simulink model "sampleModel134"  (Simulink 9.1)
settings: Solver=VariableStepAuto  StartTime=0.0  StopTime=10.0  RelTol=1e-3
undefined symbols (not defined in the file): DiscIntNeverNeededParam, Newton, Raphson
libraries: simulink x62
(part 1 of 2)
settings Model: Creator=DELL  LastModifiedBy=DELL
settings DataIOCC: SaveFormat=Dataset
settings OptimizationCC: LifeSpan=auto
settings DebuggingCC: UnderspecifiedInitializationDetection=Simplified  MergeDetectMultiDrivingBlocksExec=error  SFUnexpectedBacktrackingDiag=error  SFNoUnconditionalDefaultTransitionDiag=error  SFExecutionAtInitializationDiag=warning
settings HardwareCC: ProdBitPerPointer=64  ProdBitPerSizeT=64  ProdBitPerPtrDiffT=64  ProdLargestAtomicFloat=Float  ProdIntDivRoundTo=Zero  ProdEndianess=LittleEndian  ProdWordSize=64  ProdHWDeviceType=Intel->x86-64 (Windows64)
settings ModelReferenceCC: PropagateSignalLabelsOutOfModel=on
settings CodeAppCC: StateflowObjectComments=off
settings GRTTargetCC: TargetLangStandard=C99 (ISO)  CombineOutputUpdateFcns=on  GRTInterface=off
settings ConfigComp: CovMetricSettings=dwe  CovHtmlReporting=off  CovSaveCumulativeToWorkspaceVar=off  CovSaveSingleToWorkspaceVar=off  CovExternalEMLEnable=on

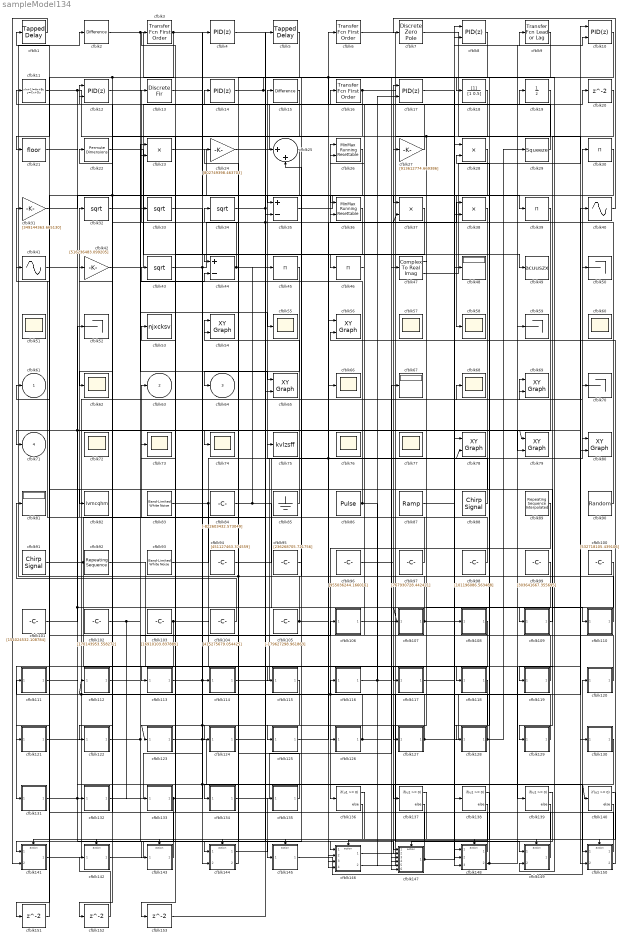
== system sampleModel134 ==
  cfblk1 : simulink/Discrete/Tapped Delay  vinit=0.0  samptime=-1  NumDelays=1  DelayOrder=Oldest  includeCurrent=off
  cfblk{8,10,12,17} (4 alike) : simulink/Continuous/PID Controller (2DOF)  Controller=PID  TimeDomain=Discrete-time  SampleTime=1  IntegratorMethod=Forward Euler  FilterMethod=Forward Euler  Form=Parallel  UseFilter=on  ControllerParametersSource=internal  P=1  I=1  D=0  N=100  b=1  c=1  InitialConditionSource=internal  InitialConditionForIntegrator=0  InitialConditionForFilter=0  ExternalReset=none  LimitOutput=off  UpperSaturationLimit=inf  LowerSaturationLimit=-inf  LinearizeAsGain=off  AntiWindupMode=none  Kb=1  TrackingMode=off  Kt=1  PParamMin=[]  PParamMax=[]  IParamMin=[]  IParamMax=[]  DParamMin=[]  DParamMax=[]  NParamMin=[]  NParamMax=[]  bParamMin=[]  bParamMax=[]  cParamMin=[]  cParamMax=[]  KbParamMin=[]  KbParamMax=[]  KtParamMin=[]  KtParamMax=[]  POutMin=[]  POutMax=[]  IOutMin=[]  IOutMax=[]  DOutMin=[]  DOutMax=[]  NOutMin=[]  NOutMax=[]  bOutMin=[]  bOutMax=[]  cOutMin=[]  cOutMax=[]  KbOutMin=[]  KbOutMax=[]  KtOutMin=[]  KtOutMax=[]  IntegratorOutMin=[]  IntegratorOutMax=[]  FilterOutMin=[]  FilterOutMax=[]  SumOutMin=[]  SumOutMax=[]  Sum1OutMin=[]  Sum1OutMax=[]  Sum2OutMin=[]  Sum2OutMax=[]  Sum3OutMin=[]  Sum3OutMax=[]  SumI1OutMin=[]  SumI1OutMax=[]  SumI2OutMin=[]  SumI2OutMax=[]  SumI3OutMin=[]  SumI3OutMax=[]  SumDOutMin=[]  SumDOutMax=[]  SaturationOutMin=[]  SaturationOutMax=[]  IntegratorContinuousStateAttributes=''  IntegratorStateMustResolveToSignalObject=off  IntegratorRTWStateStorageClass=Auto  FilterContinuousStateAttributes=''  FilterStateMustResolveToSignalObject=off  FilterRTWStateStorageClass=Auto  DifferentiatorICPrevScaledInput=0  DifferentiatorOutMin=[]  DifferentiatorOutMax=[]  FilterDiffOutCoefMin=[]  FilterDiffOutCoefMax=[]  SumDenOutMin=[]  SumDenOutMax=[]  SumNumOutMin=[]  SumNumOutMax=[]  ReciprocalOutMin=[]  ReciprocalOutMax=[]  DivideOutMin=[]  DivideOutMax=[]  TunerSelectOption=Transfer Function Based (PID Tuner App)
  cfblk100 : Constant  Value=[532718105.439106]  SampleTime=1
  cfblk101 : Constant  Value=[154024532.108784]  SampleTime=1
  cfblk102 : Constant  Value=[170143953.558272]  SampleTime=1
  cfblk103 : Constant  Value=[16910103.837889]  SampleTime=1
  cfblk104 : Constant  Value=[415275679.054425]  SampleTime=1
  cfblk105 : Constant  Value=[-179627298.961863]  SampleTime=1
  cfblk106 : Subsystem
  cfblk107 : Subsystem
  cfblk108 : Subsystem
  cfblk109 : Subsystem
  cfblk11 : DiscreteStateSpace
  cfblk110 : Subsystem
  cfblk111 : Subsystem
  cfblk112 : Subsystem
  cfblk113 : Subsystem
  cfblk114 : Subsystem
  cfblk115 : Subsystem
  cfblk116 : Subsystem
  cfblk117 : Subsystem
  cfblk118 : Subsystem
  cfblk119 : Subsystem
  cfblk120 : Subsystem
  cfblk121 : Subsystem
  cfblk122 : Subsystem
  cfblk123 : Subsystem
  cfblk124 : Subsystem
  cfblk125 : Subsystem
  cfblk126 : Subsystem
  cfblk127 : Subsystem
  cfblk128 : Subsystem
  cfblk129 : Subsystem
  cfblk13 : DiscreteFir  SampleTime=1
  cfblk130 : Subsystem
  cfblk131 : Subsystem
  cfblk132 : Subsystem
  cfblk133 : Subsystem
  cfblk134 : Subsystem
  cfblk135 : Subsystem
  cfblk{136..140} (5 alike) : If  IfExpression=u1 >= 0  SampleTime=1
  cfblk14 : simulink/Continuous/PID Controller  Controller=PID  TimeDomain=Discrete-time  SampleTime=1  IntegratorMethod=Forward Euler  FilterMethod=Forward Euler  Form=Parallel  UseFilter=on  ControllerParametersSource=internal  P=1  I=1  D=0  N=100  InitialConditionSource=internal  InitialConditionForIntegrator=0  InitialConditionForFilter=0  ExternalReset=none  LimitOutput=off  UpperSaturationLimit=inf  LowerSaturationLimit=-inf  LinearizeAsGain=off  AntiWindupMode=none  Kb=1  TrackingMode=off  Kt=1  PParamMin=[]  PParamMax=[]  IParamMin=[]  IParamMax=[]  DParamMin=[]  DParamMax=[]  NParamMin=[]  NParamMax=[]  KbParamMin=[]  KbParamMax=[]  KtParamMin=[]  KtParamMax=[]  POutMin=[]  POutMax=[]  IOutMin=[]  IOutMax=[]  DOutMin=[]  DOutMax=[]  NOutMin=[]  NOutMax=[]  KbOutMin=[]  KbOutMax=[]  KtOutMin=[]  KtOutMax=[]  IntegratorOutMin=[]  IntegratorOutMax=[]  FilterOutMin=[]  FilterOutMax=[]  SumOutMin=[]  SumOutMax=[]  SumI1OutMin=[]  SumI1OutMax=[]  SumI2OutMin=[]  SumI2OutMax=[]  SumI3OutMin=[]  SumI3OutMax=[]  SumDOutMin=[]  SumDOutMax=[]  SaturationOutMin=[]  SaturationOutMax=[]  IntegratorContinuousStateAttributes=''  IntegratorStateMustResolveToSignalObject=off  IntegratorRTWStateStorageClass=Auto  FilterContinuousStateAttributes=''  FilterStateMustResolveToSignalObject=off  FilterRTWStateStorageClass=Auto  DifferentiatorICPrevScaledInput=0  DifferentiatorOutMin=[]  DifferentiatorOutMax=[]  FilterDiffOutCoefMin=[]  FilterDiffOutCoefMax=[]  SumDenOutMin=[]  SumDenOutMax=[]  SumNumOutMin=[]  SumNumOutMax=[]  ReciprocalOutMin=[]  ReciprocalOutMax=[]  DivideOutMin=[]  DivideOutMax=[]  TunerSelectOption=Transfer Function Based (PID Tuner App)
  cfblk141 : Subsystem  TreatAsAtomicUnit=on
  cfblk142 : Subsystem  TreatAsAtomicUnit=on
  cfblk143 : Subsystem  TreatAsAtomicUnit=on
  cfblk144 : Subsystem  TreatAsAtomicUnit=on
  cfblk145 : Subsystem  TreatAsAtomicUnit=on
  cfblk146 : Subsystem  TreatAsAtomicUnit=on
  cfblk147 : Subsystem  TreatAsAtomicUnit=on
  cfblk148 : Subsystem  TreatAsAtomicUnit=on
  cfblk149 : Subsystem  TreatAsAtomicUnit=on
  cfblk15 : simulink/Discrete/Difference  ICPrevInput=0.0  OutMin=[]  OutMax=[]  OutDataTypeStr=Inherit: Inherit via back propagation  OutDataType=fixdt(1, 16)  OutScaling=2^-10  DoSatur=off
  cfblk150 : Subsystem  TreatAsAtomicUnit=on
  cfblk{20,151..153} (4 alike) : Delay  SampleTime=1
  cfblk16 : simulink/Discrete/Transfer Fcn First Order  PoleZ=0.95  ICPrevOutput=0.0  DoSatur=off
      settings: SourceProductName=Simulink
  cfblk18 : DiscreteFilter  SampleTime=1
  cfblk19 : UnitDelay
  cfblk2 : simulink/Discrete/Difference  ICPrevInput=0.0  OutMin=[]  OutMax=[]  OutDataTypeStr=Inherit: Inherit via back propagation  OutDataType=fixdt(1, 16)  OutScaling=2^-10  DoSatur=off
  cfblk21 : Rounding
  cfblk22 : PermuteDimensions
  cfblk23 : Product  Inputs=**
  cfblk24 : Gain  Gain=[802749398.463703]
  cfblk25 : Sum  Inputs=|++
  cfblk26 : simulink/Math Operations/MinMax Running Resettable  Function=min  vinit=0.0
  cfblk27 : Gain  Gain=[913612774.669386]
  cfblk28 : Product
  cfblk29 : Squeeze
  cfblk3 : simulink/Discrete/Transfer Fcn First Order  PoleZ=0.95  ICPrevOutput=0.0  DoSatur=off
      settings: SourceProductName=Simulink
  cfblk{30,39,45..46} (4 alike) : Product  Inputs=*
  cfblk31 : Gain  Gain=[349144363.665130]
  cfblk{32..34,43} (4 alike) : Sqrt  SaturateOnIntegerOverflow=on
  cfblk35 : Sum  Inputs=+-
  cfblk36 : simulink/Math Operations/MinMax Running Resettable  Function=min  vinit=0.0
  cfblk37 : Product
  cfblk38 : Product
  cfblk4 : simulink/Continuous/PID Controller  Controller=PID  TimeDomain=Discrete-time  SampleTime=1  IntegratorMethod=Forward Euler  FilterMethod=Forward Euler  Form=Parallel  UseFilter=on  ControllerParametersSource=internal  P=1  I=1  D=0  N=100  InitialConditionSource=internal  InitialConditionForIntegrator=0  InitialConditionForFilter=0  ExternalReset=none  LimitOutput=off  UpperSaturationLimit=inf  LowerSaturationLimit=-inf  LinearizeAsGain=off  AntiWindupMode=none  Kb=1  TrackingMode=off  Kt=1  PParamMin=[]  PParamMax=[]  IParamMin=[]  IParamMax=[]  DParamMin=[]  DParamMax=[]  NParamMin=[]  NParamMax=[]  KbParamMin=[]  KbParamMax=[]  KtParamMin=[]  KtParamMax=[]  POutMin=[]  POutMax=[]  IOutMin=[]  IOutMax=[]  DOutMin=[]  DOutMax=[]  NOutMin=[]  NOutMax=[]  KbOutMin=[]  KbOutMax=[]  KtOutMin=[]  KtOutMax=[]  IntegratorOutMin=[]  IntegratorOutMax=[]  FilterOutMin=[]  FilterOutMax=[]  SumOutMin=[]  SumOutMax=[]  SumI1OutMin=[]  SumI1OutMax=[]  SumI2OutMin=[]  SumI2OutMax=[]  SumI3OutMin=[]  SumI3OutMax=[]  SumDOutMin=[]  SumDOutMax=[]  SaturationOutMin=[]  SaturationOutMax=[]  IntegratorContinuousStateAttributes=''  IntegratorStateMustResolveToSignalObject=off  IntegratorRTWStateStorageClass=Auto  FilterContinuousStateAttributes=''  FilterStateMustResolveToSignalObject=off  FilterRTWStateStorageClass=Auto  DifferentiatorICPrevScaledInput=0  DifferentiatorOutMin=[]  DifferentiatorOutMax=[]  FilterDiffOutCoefMin=[]  FilterDiffOutCoefMax=[]  SumDenOutMin=[]  SumDenOutMax=[]  SumNumOutMin=[]  SumNumOutMax=[]  ReciprocalOutMin=[]  ReciprocalOutMax=[]  DivideOutMin=[]  DivideOutMax=[]  TunerSelectOption=Transfer Function Based (PID Tuner App)
  cfblk40 : Sin  TimeSource=Use external signal  SampleTime=0
  cfblk41 : Sin  TimeSource=Use external signal  SampleTime=0
  cfblk42 : Gain  Gain=[516236483.099205]
  cfblk44 : Sum  Inputs=+-
  cfblk47 : ComplexToRealImag
  cfblk48 : Display
  cfblk49 : ToWorkspace  VariableName=acuuszx  SaveFormat=Timeseries  SampleTime=-1
  cfblk5 : simulink/Discrete/Tapped Delay  vinit=0.0  samptime=-1  NumDelays=1  DelayOrder=Oldest  includeCurrent=off
  cfblk{50,52,59,70} (4 alike) : Terminator
  cfblk{51,55,57..58,60,62,66,68,72..74,76..77} (13 alike) : Scope
      cfblk51 settings: Floating=on
      cfblk57 settings: Floating=on
      cfblk60 settings: Floating=on
      cfblk72 settings: Floating=on
      cfblk76 settings: Floating=on
      cfblk77 settings: Floating=on
  cfblk53 : ToWorkspace  VariableName=njxcksv  SaveFormat=Timeseries  SampleTime=-1
  cfblk{54,56,65,69,78..80} (7 alike) : simulink/Sinks/XY Graph  xmin=-1  xmax=1  ymin=-1  ymax=1  st=-1
  cfblk6 : simulink/Discrete/Transfer Fcn First Order  PoleZ=0.95  ICPrevOutput=0.0  DoSatur=off
      settings: SourceProductName=Simulink
  cfblk67 : Display
  cfblk7 : DiscreteZeroPole  Poles=[0 0.5]  Gain=1
  cfblk75 : ToWorkspace  VariableName=kvlzsff  SaveFormat=Timeseries  SampleTime=-1
  cfblk81 : Display
  cfblk82 : ToWorkspace  VariableName=lvmcqhm  SaveFormat=Timeseries  SampleTime=-1
  cfblk83 : simulink/Sources/Band-Limited White Noise  Cov=[8169729141.864307]  Ts=0.1  seed=[2785039100.000000]
  cfblk84 : Constant  Value=[-822603432.573049]  SampleTime=1
  cfblk85 : Ground
  cfblk86 : DiscretePulseGenerator  PulseType=Time based  Amplitude=[750082267.243392]  Period=[37122237.282737]  PulseWidth=5  PhaseDelay=[9.000000]
  cfblk87 : simulink/Sources/Ramp  slope=[-5292.833799]  start=[18.154667]  InitialOutput=[974234.405422]
  cfblk88 : simulink/Sources/Chirp Signal  f1=[-748836999.070379]  T=[-805840635.110502]  f2=[-105823570.334951]
  cfblk89 : simulink/Sources/Repeating Sequence Interpolated  OutValues=[705421503.917708, -895308717.922875, -981590852.788041, 588384265.742355, 525308445.664458]  TimeValues=[0 0.1 0.5 0.6 1].'  LookUpMeth=Use Input Nearest  tsamp=0.01  OutMin=[]  OutMax=[]  OutDataTypeStr=double  OutputDataTypeScalingMode=double  OutDataType=fixdt(0,8)  OutScaling=2^-10
  cfblk9 : simulink/Discrete/Transfer Fcn Lead or Lag  PoleZ=0.95  ZeroZ=0.75  ICPrevOutput=0.0  ICPrevInput=0.0  DoSatur=off
      settings: SourceProductName=Simulink  SourceProductBaseCode=SL
  cfblk90 : UniformRandomNumber  Minimum=[-9644754940.784754]  Maximum=[7557952401.651167]  Seed=[38216483.000000]  SampleTime=0.1
  cfblk91 : simulink/Sources/Chirp Signal  f1=[518839843.170434]  T=[500119055.611744]  f2=[-520193458.683903]
  cfblk92 : simulink/Sources/Repeating Sequence  rep_seq_t=[0 2]  rep_seq_y=[-918028262.635120, -492802667.715167]
  cfblk93 : simulink/Sources/Band-Limited White Noise  Cov=[2518627408.787849]  Ts=0.1  seed=[317239943.000000]
  cfblk94 : Constant  Value=[451127463.374559]  SampleTime=1
  cfblk95 : Constant  Value=[236268705.721756]  SampleTime=1
  cfblk96 : Constant  Value=[955036244.166016]  SampleTime=1
  cfblk97 : Constant  Value=[767930728.442421]  SampleTime=1
  cfblk98 : Constant  Value=[101196086.563488]  SampleTime=1
  cfblk99 : Constant  Value=[303641667.355695]  SampleTime=1
  cfblk61 : Outport
  cfblk63 : Outport  Port=2
  cfblk64 : Outport  Port=3
  cfblk71 : Outport  Port=4
  wires:
  cfblk22/1 -> cfblk46/1
  cfblk45/1 -> cfblk64/1
  cfblk83/1 -> cfblk15/1, cfblk150/2(cfblk13)
  cfblk89/1 -> cfblk136/1
  cfblk106/1(cfblk2) -> cfblk149/1(cfblk1)
  cfblk109/1(cfblk2) -> cfblk32/1
  cfblk145/1(cfblk2) -> cfblk120/1(cfblk1)
  cfblk14/1 -> cfblk149/2(cfblk13), cfblk79/2
  cfblk31/1 -> cfblk39/1
  cfblk3/1 -> cfblk62/1, cfblk21/1, cfblk38/2
  cfblk9/1 -> cfblk74/1
  cfblk105/1 -> cfblk78/2, cfblk38/1, cfblk2/1
  cfblk20/1 -> cfblk119/1(cfblk1)
  cfblk27/1 -> cfblk14/1
  cfblk44/1 -> cfblk12/1, cfblk109/1(cfblk1)
  cfblk95/1 -> cfblk141/1(cfblk1)
  cfblk28/1 -> cfblk151/1, cfblk152/1
  cfblk148/1(cfblk2) -> cfblk34/1
  cfblk104/1 -> cfblk81/1
  cfblk23/1 -> cfblk58/1
  cfblk6/1 -> cfblk118/1(cfblk1)
  cfblk113/1(cfblk2) -> cfblk114/1(cfblk1), cfblk19/1
  cfblk130/1(cfblk2) -> cfblk134/1(cfblk1)
  cfblk121/1(cfblk2) -> cfblk30/1, cfblk78/1
  cfblk143/1(cfblk2) -> cfblk22/1
  cfblk32/1 -> cfblk13/1
  cfblk96/1 -> cfblk17/1
  cfblk98/1 -> cfblk31/1
  cfblk119/1(cfblk2) -> cfblk16/1
  cfblk43/1 -> cfblk26/1, cfblk146/4(cfblk16)
  cfblk24/1 -> cfblk6/1
  cfblk40/1 -> cfblk7/1
  cfblk108/1(cfblk2) -> cfblk131/1(cfblk1)
  cfblk123/1(cfblk2) -> cfblk150/1(cfblk1), cfblk69/1
  cfblk36/1 -> cfblk44/1
  cfblk146/1(cfblk2) -> cfblk27/1
  cfblk88/1 -> cfblk75/1
  cfblk148/2(cfblk17) -> cfblk112/1(cfblk1), cfblk116/1(cfblk1), cfblk10/2
  cfblk115/1(cfblk2) -> cfblk123/1(cfblk1), cfblk144/2(cfblk14)
  cfblk2/1 -> cfblk47/1, cfblk55/1
  cfblk117/1(cfblk2) -> cfblk9/1
  cfblk19/1 -> cfblk117/1(cfblk1), cfblk147/3(cfblk6)
  cfblk120/1(cfblk2) -> cfblk61/1
  cfblk146/2(cfblk17) -> cfblk40/1
  cfblk150/1(cfblk2) -> cfblk111/1(cfblk1)
  cfblk127/1(cfblk2) -> cfblk59/1, cfblk41/1
  cfblk114/1(cfblk2) -> cfblk50/1
  cfblk135/1(cfblk2) -> cfblk24/1
  cfblk10/1 -> cfblk128/1(cfblk1)
  cfblk35/1 -> cfblk37/1
  cfblk47/1 -> cfblk125/1(cfblk1)
  cfblk141/1(cfblk2) -> cfblk28/1
  cfblk5/1 -> cfblk124/1(cfblk1)
  cfblk99/1 -> cfblk127/1(cfblk1)
  cfblk85/1 -> cfblk54/1
  cfblk33/1 -> cfblk49/1
  cfblk93/1 -> cfblk8/1
  cfblk7/1 -> cfblk130/1(cfblk1)
  cfblk147/1(cfblk2) -> cfblk53/1, cfblk80/1
  cfblk133/1(cfblk2) -> cfblk140/1, cfblk20/1, cfblk143/1(cfblk1)
  cfblk26/1 -> cfblk35/1
  cfblk39/1 -> cfblk71/1
  cfblk13/1 -> cfblk18/1
  cfblk129/1(cfblk2) -> cfblk28/2
  cfblk18/1 -> cfblk113/1(cfblk1)
  cfblk103/1 -> cfblk148/1(cfblk1), cfblk122/1(cfblk1)
  cfblk1/1 -> cfblk141/2(cfblk10)
  cfblk21/1 -> cfblk79/1, cfblk147/4(cfblk7)
  cfblk30/1 -> cfblk36/1
  cfblk97/1 -> cfblk63/1
  cfblk142/1(cfblk2) -> cfblk146/1(cfblk1)
  cfblk15/1 -> cfblk82/1
  cfblk38/1 -> cfblk121/1(cfblk1)
  cfblk12/1 -> cfblk65/1
  cfblk100/1 -> cfblk129/1(cfblk1)
  cfblk11/1 -> cfblk107/1(cfblk1), cfblk146/2(cfblk14), cfblk56/1
  cfblk47/2 -> cfblk10/1
  cfblk107/1(cfblk2) -> cfblk108/1(cfblk1), cfblk25/2
  cfblk25/1 -> cfblk35/2
  cfblk134/1(cfblk2) -> cfblk67/1
  cfblk90/1 -> cfblk36/2
  cfblk84/1 -> cfblk110/1(cfblk1), cfblk45/1
  cfblk29/1 -> cfblk11/1
  cfblk126/1(cfblk2) -> cfblk73/1, cfblk69/2
  cfblk110/1(cfblk2) -> cfblk42/1, cfblk54/2
  cfblk116/1(cfblk2) -> cfblk68/1, cfblk17/2
  cfblk132/1(cfblk2) -> cfblk4/1
  cfblk42/1 -> cfblk8/2
  cfblk94/1 -> cfblk70/1
  cfblk149/1(cfblk2) -> cfblk12/2
  cfblk101/1 -> cfblk52/1
  cfblk102/1 -> cfblk23/1, cfblk133/1(cfblk1)
  cfblk144/1(cfblk2) -> cfblk135/1(cfblk1)
  cfblk144/2(cfblk15) -> cfblk33/1
  cfblk128/1(cfblk2) -> cfblk3/1, cfblk29/1
  cfblk131/1(cfblk2) -> cfblk23/2
  cfblk122/1(cfblk2) -> cfblk44/2, cfblk145/1(cfblk1)
  cfblk124/1(cfblk2) -> cfblk147/1(cfblk1)
  cfblk112/1(cfblk2) -> cfblk106/1(cfblk1)
  cfblk125/1(cfblk2) -> cfblk66/1
  cfblk46/1 -> cfblk26/2
  cfblk111/1(cfblk2) -> cfblk137/1
  cfblk17/1 -> cfblk138/1
  cfblk91/1 -> cfblk65/2, cfblk139/1
  cfblk34/1 -> cfblk80/2, cfblk37/2, cfblk5/1
  cfblk150/2(cfblk14) -> cfblk56/2
  cfblk92/1 -> cfblk126/1(cfblk1)
  cfblk16/1 -> cfblk148/2(cfblk15), cfblk144/1(cfblk1)
  cfblk41/1 -> cfblk132/1(cfblk1), cfblk147/6(cfblk9)
  cfblk87/1 -> cfblk48/1
  cfblk4/1 -> cfblk147/2(cfblk5)
  cfblk8/1 -> cfblk115/1(cfblk1), cfblk146/3(cfblk15)
  cfblk86/1 -> cfblk43/1, cfblk147/5(cfblk8)
  cfblk118/1(cfblk2) -> cfblk148/3(cfblk16)
  cfblk136/1 -> cfblk141/Action
  cfblk136/2 -> cfblk142/Action
  cfblk137/1 -> cfblk143/Action
  cfblk137/2 -> cfblk144/Action
  cfblk138/1 -> cfblk145/Action
  cfblk138/2 -> cfblk146/Action
  cfblk139/1 -> cfblk147/Action
  cfblk139/2 -> cfblk148/Action
  cfblk140/1 -> cfblk149/Action
  cfblk140/2 -> cfblk150/Action
  cfblk151/1 -> cfblk1/1
  cfblk152/1 -> cfblk142/1(cfblk1)
  cfblk37/1 -> cfblk153/1
  cfblk153/1 -> cfblk25/1

== system sampleModel134/cfblk106 ==
  cfblk1 : Inport
  cfblk2 : Outport
  wires:
  cfblk1/1 -> cfblk2/1

== system sampleModel134/cfblk107 ==
  cfblk1 : Inport
  cfblk2 : Outport
  wires:
  cfblk1/1 -> cfblk2/1

== system sampleModel134/cfblk108 ==
  cfblk1 : Inport
  cfblk2 : Outport
  wires:
  cfblk1/1 -> cfblk2/1

== system sampleModel134/cfblk109 ==
  cfblk1 : Inport
  cfblk2 : Outport
  wires:
  cfblk1/1 -> cfblk2/1

== system sampleModel134/cfblk110 ==
  cfblk1 : Inport
  cfblk2 : Outport
  wires:
  cfblk1/1 -> cfblk2/1

== system sampleModel134/cfblk111 ==
  cfblk1 : Inport
  cfblk2 : Outport
  wires:
  cfblk1/1 -> cfblk2/1

== system sampleModel134/cfblk112 ==
  cfblk1 : Inport
  cfblk2 : Outport
  wires:
  cfblk1/1 -> cfblk2/1

== system sampleModel134/cfblk113 ==
  cfblk1 : Inport
  cfblk2 : Outport
  wires:
  cfblk1/1 -> cfblk2/1

== system sampleModel134/cfblk114 ==
  cfblk1 : Inport
  cfblk2 : Outport
  wires:
  cfblk1/1 -> cfblk2/1

== system sampleModel134/cfblk115 ==
  cfblk1 : Inport
  cfblk2 : Outport
  wires:
  cfblk1/1 -> cfblk2/1

== system sampleModel134/cfblk116 ==
  cfblk1 : Inport
  cfblk2 : Outport
  wires:
  cfblk1/1 -> cfblk2/1

== system sampleModel134/cfblk117 ==
  cfblk1 : Inport
  cfblk2 : Outport
  wires:
  cfblk1/1 -> cfblk2/1

== system sampleModel134/cfblk118 ==
  cfblk1 : Inport
  cfblk2 : Outport
  wires:
  cfblk1/1 -> cfblk2/1

== system sampleModel134/cfblk119 ==
  cfblk1 : Inport
  cfblk2 : Outport
  wires:
  cfblk1/1 -> cfblk2/1

== system sampleModel134/cfblk120 ==
  cfblk1 : Inport
  cfblk2 : Outport
  wires:
  cfblk1/1 -> cfblk2/1

== system sampleModel134/cfblk121 ==
  cfblk1 : Inport
  cfblk2 : Outport
  wires:
  cfblk1/1 -> cfblk2/1

== system sampleModel134/cfblk122 ==
  cfblk1 : Inport
  cfblk2 : Outport
  wires:
  cfblk1/1 -> cfblk2/1

== system sampleModel134/cfblk123 ==
  cfblk1 : Inport
  cfblk2 : Outport
  wires:
  cfblk1/1 -> cfblk2/1

== system sampleModel134/cfblk124 ==
  cfblk1 : Inport
  cfblk2 : Outport
  wires:
  cfblk1/1 -> cfblk2/1

== system sampleModel134/cfblk125 ==
  cfblk1 : Inport
  cfblk2 : Outport
  wires:
  cfblk1/1 -> cfblk2/1

== system sampleModel134/cfblk126 ==
  cfblk1 : Inport
  cfblk2 : Outport
  wires:
  cfblk1/1 -> cfblk2/1

== system sampleModel134/cfblk127 ==
  cfblk1 : Inport
  cfblk2 : Outport
  wires:
  cfblk1/1 -> cfblk2/1

== system sampleModel134/cfblk128 ==
  cfblk1 : Inport
  cfblk2 : Outport
  wires:
  cfblk1/1 -> cfblk2/1

== system sampleModel134/cfblk129 ==
  cfblk1 : Inport
  cfblk2 : Outport
  wires:
  cfblk1/1 -> cfblk2/1

== system sampleModel134/cfblk130 ==
  cfblk1 : Inport
  cfblk2 : Outport
  wires:
  cfblk1/1 -> cfblk2/1

== system sampleModel134/cfblk131 ==
  cfblk1 : Inport
  cfblk2 : Outport
  wires:
  cfblk1/1 -> cfblk2/1

== system sampleModel134/cfblk132 ==
  cfblk1 : Inport
  cfblk2 : Outport
  wires:
  cfblk1/1 -> cfblk2/1

== system sampleModel134/cfblk133 ==
  cfblk1 : Inport
  cfblk2 : Outport
  wires:
  cfblk1/1 -> cfblk2/1

== system sampleModel134/cfblk134 ==
  cfblk1 : Inport
  cfblk2 : Outport
  wires:
  cfblk1/1 -> cfblk2/1

== system sampleModel134/cfblk135 ==
  cfblk1 : Inport
  cfblk2 : Outport
  wires:
  cfblk1/1 -> cfblk2/1

== system sampleModel134/cfblk141 ==
  cfblk1 : Inport
  cfblk10 : Inport  Port=2
  Action Port : ActionPort  ActionType=then
  cfblk11 : Subsystem  TreatAsAtomicUnit=on
  cfblk12 : Subsystem  TreatAsAtomicUnit=on
  cfblk13 : Delay
  cfblk14 : Delay
  cfblk3 : Gain  Gain=[634647826.023846]
  cfblk4 : Signum
  cfblk5 : Subsystem
  cfblk6 : Subsystem
  cfblk7 : Subsystem
  cfblk8 : Subsystem
  cfblk9 : If  IfExpression=u1 >= 0  SampleTime=1
  cfblk2 : Outport
  wires:
  cfblk12/1(cfblk2) -> cfblk7/1(cfblk1)
  cfblk10/1 -> cfblk3/1
  cfblk3/1 -> cfblk12/1(cfblk1)
  cfblk5/1(cfblk2) -> cfblk4/1
  cfblk6/1(cfblk2) -> cfblk11/1(cfblk1)
  cfblk11/1(cfblk2) -> cfblk5/1(cfblk1)
  cfblk1/1 -> cfblk6/1(cfblk1)
  cfblk8/1(cfblk2) -> cfblk2/1
  cfblk11/2(cfblk9) -> cfblk8/1(cfblk1)
  cfblk9/1 -> cfblk11/Action
  cfblk9/2 -> cfblk12/Action
  cfblk4/1 -> cfblk13/1
  cfblk13/1 -> cfblk9/1
  cfblk7/1(cfblk2) -> cfblk14/1
  cfblk14/1 -> cfblk12/2(cfblk8)

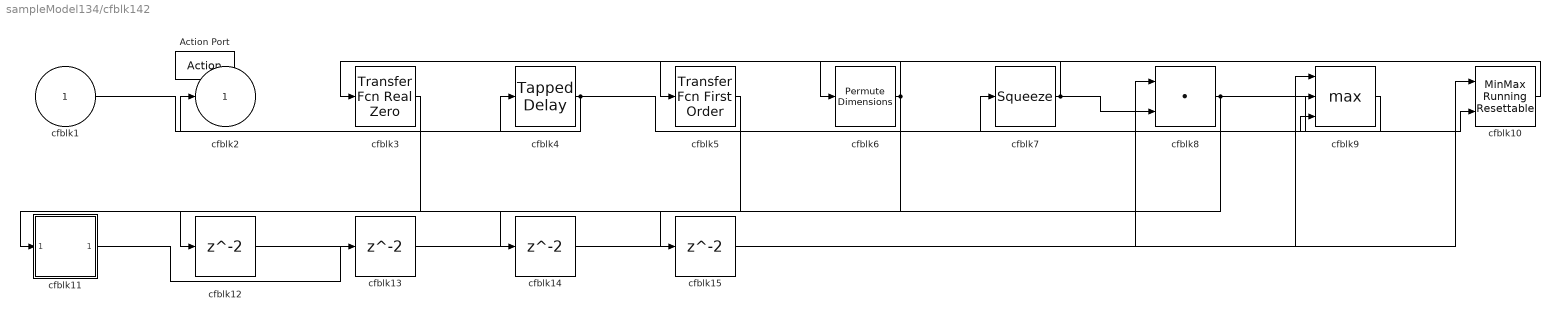
== system sampleModel134/cfblk142 ==
  cfblk1 : Inport
  Action Port : ActionPort  ActionType=else
  cfblk10 : simulink/Math Operations/MinMax Running Resettable  Function=min  vinit=0.0
  cfblk11 : Subsystem
  cfblk{12..15} (4 alike) : Delay
  cfblk3 : simulink/Discrete/Transfer Fcn Real Zero  ZeroZ=0.75  ICPrevInput=0.0  DoSatur=off
      settings: SourceProductName=Simulink  SourceProductBaseCode=SL
  cfblk4 : simulink/Discrete/Tapped Delay  vinit=0.0  samptime=-1  NumDelays=1  DelayOrder=Oldest  includeCurrent=off
  cfblk5 : simulink/Discrete/Transfer Fcn First Order  PoleZ=0.95  ICPrevOutput=0.0  DoSatur=off
      settings: SourceProductName=Simulink
  cfblk6 : PermuteDimensions
  cfblk7 : Squeeze
  cfblk8 : DotProduct  InputSameDT=on  OutDataTypeStr=Inherit: Inherit via internal rule
  cfblk9 : MinMax  Function=max  Inputs=3
  cfblk2 : Outport
  wires:
  cfblk4/1 -> cfblk2/1, cfblk9/3
  cfblk10/1 -> cfblk6/1
  cfblk9/1 -> cfblk7/1
  cfblk7/1 -> cfblk3/1, cfblk8/2
  cfblk1/1 -> cfblk4/1
  cfblk8/1 -> cfblk10/2, cfblk15/1
  cfblk5/1 -> cfblk11/1(cfblk1)
  cfblk6/1 -> cfblk5/1, cfblk14/1
  cfblk3/1 -> cfblk12/1
  cfblk12/1 -> cfblk9/1
  cfblk11/1(cfblk2) -> cfblk13/1
  cfblk13/1 -> cfblk10/1
  cfblk14/1 -> cfblk8/1
  cfblk15/1 -> cfblk9/2

== system sampleModel134/cfblk143 ==
  cfblk1 : Inport
  Action Port : ActionPort  ActionType=then
  cfblk3 : simulink/Discrete/Difference  ICPrevInput=0.0  OutMin=[]  OutMax=[]  OutDataTypeStr=Inherit: Inherit via back propagation  OutDataType=fixdt(1, 16)  OutScaling=2^-10  DoSatur=off
  cfblk4 : simulink/Discrete/Transfer Fcn Lead or Lag  PoleZ=0.95  ZeroZ=0.75  ICPrevOutput=0.0  ICPrevInput=0.0  DoSatur=off
      settings: SourceProductName=Simulink  SourceProductBaseCode=SL
  cfblk5 : DiscreteTransferFcn
  cfblk6 : Sum  Inputs=|++
  cfblk7 : Product  Inputs=*
  cfblk8 : Product  Inputs=**
  cfblk9 : Delay
  cfblk2 : Outport
  wires:
  cfblk3/1 -> cfblk6/1
  cfblk1/1 -> cfblk7/1
  cfblk5/1 -> cfblk4/1, cfblk8/1
  cfblk7/1 -> cfblk3/1, cfblk8/2
  cfblk6/1 -> cfblk5/1
  cfblk8/1 -> cfblk2/1
  cfblk4/1 -> cfblk9/1
  cfblk9/1 -> cfblk6/2

== system sampleModel134/cfblk144 ==
  cfblk1 : Inport
  cfblk14 : Inport  Port=2
  Action Port : ActionPort  ActionType=else
  cfblk10 : Constant  Value=[490207388.307763]  SampleTime=1
  cfblk11 : Subsystem
  cfblk12 : Subsystem
  cfblk13 : Subsystem
  cfblk3 : DiscreteZeroPole  Poles=[0 0.5]  Gain=1  SampleTime=-1
  cfblk4 : DiscreteStateSpace  SampleTime=-1
  cfblk5 : Delay
  cfblk6 : Sum  Inputs=-+
  cfblk7 : PermuteDimensions
  cfblk8 : Abs
  cfblk9 : Sum
  cfblk2 : Outport
  cfblk15 : Outport  Port=2
  wires:
  cfblk14/1 -> cfblk6/1
  cfblk9/1 -> cfblk6/2
  cfblk8/1 -> cfblk3/1
  cfblk7/1 -> cfblk5/1
  cfblk11/1(cfblk2) -> cfblk7/1
  cfblk12/1(cfblk2) -> cfblk8/1
  cfblk5/1 -> cfblk4/1, cfblk12/1(cfblk1)
  cfblk6/1 -> cfblk2/1
  cfblk4/1 -> cfblk13/1(cfblk1)
  cfblk10/1 -> cfblk11/1(cfblk1)
  cfblk1/1 -> cfblk15/1
  cfblk13/1(cfblk2) -> cfblk9/1
  cfblk3/1 -> cfblk9/2

== system sampleModel134/cfblk145 ==
  cfblk1 : Inport
  Action Port : ActionPort  ActionType=then
  cfblk3 : Gain  Gain=[-467909328.377413]
  cfblk4 : Subsystem
  cfblk5 : Subsystem
  cfblk6 : Subsystem
  cfblk7 : Subsystem
  cfblk2 : Outport
  wires:
  cfblk5/1(cfblk2) -> cfblk3/1
  cfblk1/1 -> cfblk5/1(cfblk1)
  cfblk7/1(cfblk2) -> cfblk2/1
  cfblk6/1(cfblk2) -> cfblk4/1(cfblk1)
  cfblk4/1(cfblk2) -> cfblk7/1(cfblk1)
  cfblk3/1 -> cfblk6/1(cfblk1)

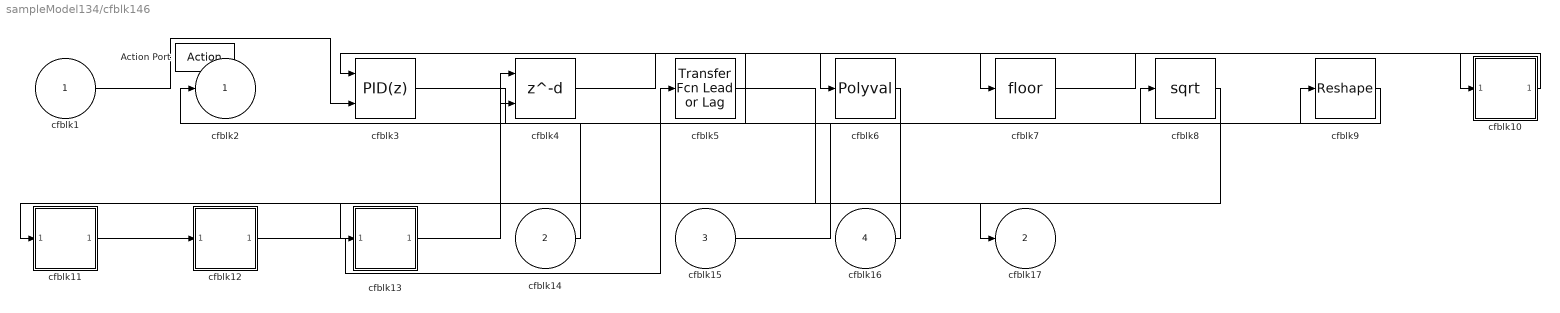
== system sampleModel134/cfblk146 ==
  cfblk1 : Inport
  cfblk14 : Inport  Port=2
  cfblk15 : Inport  Port=3
  cfblk16 : Inport  Port=4
  Action Port : ActionPort  ActionType=else
  cfblk10 : Subsystem
  cfblk11 : Subsystem
  cfblk12 : Subsystem
  cfblk13 : Subsystem
  cfblk3 : simulink/Continuous/PID Controller (2DOF)  Controller=PID  TimeDomain=Discrete-time  SampleTime=-1  IntegratorMethod=Forward Euler  FilterMethod=Forward Euler  Form=Parallel  UseFilter=on  ControllerParametersSource=internal  P=1  I=1  D=0  N=100  b=1  c=1  InitialConditionSource=internal  InitialConditionForIntegrator=0  InitialConditionForFilter=0  ExternalReset=none  LimitOutput=off  UpperSaturationLimit=inf  LowerSaturationLimit=-inf  LinearizeAsGain=off  AntiWindupMode=none  Kb=1  TrackingMode=off  Kt=1  PParamMin=[]  PParamMax=[]  IParamMin=[]  IParamMax=[]  DParamMin=[]  DParamMax=[]  NParamMin=[]  NParamMax=[]  bParamMin=[]  bParamMax=[]  cParamMin=[]  cParamMax=[]  KbParamMin=[]  KbParamMax=[]  KtParamMin=[]  KtParamMax=[]  POutMin=[]  POutMax=[]  IOutMin=[]  IOutMax=[]  DOutMin=[]  DOutMax=[]  NOutMin=[]  NOutMax=[]  bOutMin=[]  bOutMax=[]  cOutMin=[]  cOutMax=[]  KbOutMin=[]  KbOutMax=[]  KtOutMin=[]  KtOutMax=[]  IntegratorOutMin=[]  IntegratorOutMax=[]  FilterOutMin=[]  FilterOutMax=[]  SumOutMin=[]  SumOutMax=[]  Sum1OutMin=[]  Sum1OutMax=[]  Sum2OutMin=[]  Sum2OutMax=[]  Sum3OutMin=[]  Sum3OutMax=[]  SumI1OutMin=[]  SumI1OutMax=[]  SumI2OutMin=[]  SumI2OutMax=[]  SumI3OutMin=[]  SumI3OutMax=[]  SumDOutMin=[]  SumDOutMax=[]  SaturationOutMin=[]  SaturationOutMax=[]  IntegratorContinuousStateAttributes=''  IntegratorStateMustResolveToSignalObject=off  IntegratorRTWStateStorageClass=Auto  FilterContinuousStateAttributes=''  FilterStateMustResolveToSignalObject=off  FilterRTWStateStorageClass=Auto  DifferentiatorICPrevScaledInput=0  DifferentiatorOutMin=[]  DifferentiatorOutMax=[]  FilterDiffOutCoefMin=[]  FilterDiffOutCoefMax=[]  SumDenOutMin=[]  SumDenOutMax=[]  SumNumOutMin=[]  SumNumOutMax=[]  ReciprocalOutMin=[]  ReciprocalOutMax=[]  DivideOutMin=[]  DivideOutMax=[]  TunerSelectOption=Transfer Function Based (PID Tuner App)
  cfblk4 : Delay  DelayLengthSource=Input port
      settings: InputPortMap=u0,p1
  cfblk5 : simulink/Discrete/Transfer Fcn Lead or Lag  PoleZ=0.95  ZeroZ=0.75  ICPrevOutput=0.0  ICPrevInput=0.0  DoSatur=off
      settings: SourceProductName=Simulink  SourceProductBaseCode=SL
  cfblk6 : Polyval  Coefs=[ +2.081618890e-019, -1.441693666e-014, +4.719686976e-010, -8.536869453e-006, +1.621573104e-001, -8.087801117e+001 ]
  cfblk7 : Rounding
  cfblk8 : Sqrt  SaturateOnIntegerOverflow=on
  cfblk9 : Reshape
  cfblk2 : Outport
  cfblk17 : Outport  Port=2
  wires:
  cfblk14/1 -> cfblk2/1
  cfblk10/1(cfblk2) -> cfblk6/1
  cfblk12/1(cfblk2) -> cfblk5/1
  cfblk11/1(cfblk2) -> cfblk12/1(cfblk1)
  cfblk13/1(cfblk2) -> cfblk4/1
  cfblk16/1 -> cfblk3/1
  cfblk3/1 -> cfblk9/1
  cfblk9/1 -> cfblk4/2
  cfblk15/1 -> cfblk8/1
  cfblk1/1 -> cfblk3/2
  cfblk6/1 -> cfblk11/1(cfblk1)
  cfblk5/1 -> cfblk17/1
  cfblk4/1 -> cfblk7/1
  cfblk7/1 -> cfblk10/1(cfblk1)
  cfblk8/1 -> cfblk13/1(cfblk1)

== system sampleModel134/cfblk147 ==
  cfblk1 : Inport
  cfblk5 : Inport  Port=2
  cfblk6 : Inport  Port=3
  cfblk7 : Inport  Port=4
  cfblk8 : Inport  Port=5
  cfblk9 : Inport  Port=6
  Action Port : ActionPort  ActionType=then
  cfblk3 : DiscreteFir
  cfblk4 : Subsystem
  cfblk2 : Outport
  wires:
  cfblk6/1 -> cfblk3/1
  cfblk3/1 -> cfblk4/1(cfblk1)
  cfblk9/1 -> cfblk2/1

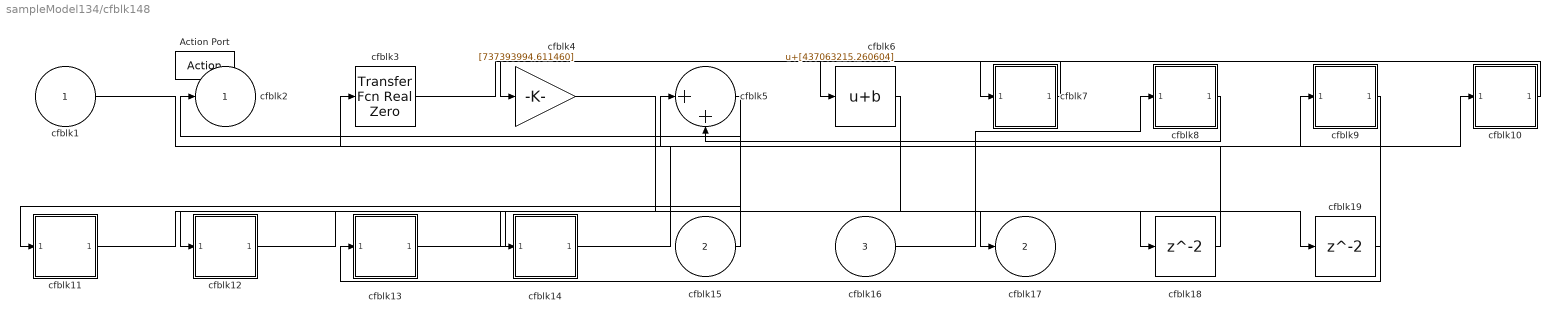
== system sampleModel134/cfblk148 ==
  cfblk1 : Inport
  cfblk15 : Inport  Port=2
  cfblk16 : Inport  Port=3
  Action Port : ActionPort  ActionType=else
  cfblk10 : Subsystem
  cfblk11 : Subsystem
  cfblk12 : Subsystem
  cfblk13 : Subsystem
  cfblk14 : Subsystem
  cfblk18 : Delay
  cfblk19 : Delay
  cfblk3 : simulink/Discrete/Transfer Fcn Real Zero  ZeroZ=0.75  ICPrevInput=0.0  DoSatur=off
      settings: SourceProductName=Simulink  SourceProductBaseCode=SL
  cfblk4 : Gain  Gain=[737393994.611460]
  cfblk5 : Sum  Inputs=|++
  cfblk6 : Bias  Bias=[437063215.260604]
  cfblk7 : Subsystem
  cfblk8 : Subsystem
  cfblk9 : Subsystem
  cfblk2 : Outport
  cfblk17 : Outport  Port=2
  wires:
  cfblk13/1(cfblk2) -> cfblk17/1
  cfblk7/1(cfblk2) -> cfblk4/1
  cfblk5/1 -> cfblk11/1(cfblk1)
  cfblk3/1 -> cfblk7/1(cfblk1)
  cfblk15/1 -> cfblk2/1
  cfblk6/1 -> cfblk12/1(cfblk1)
  cfblk9/1(cfblk2) -> cfblk13/1(cfblk1)
  cfblk11/1(cfblk2) -> cfblk14/1(cfblk1)
  cfblk16/1 -> cfblk8/1(cfblk1)
  cfblk10/1(cfblk2) -> cfblk6/1
  cfblk8/1(cfblk2) -> cfblk5/2
  cfblk1/1 -> cfblk9/1(cfblk1)
  cfblk14/1(cfblk2) -> cfblk10/1(cfblk1)
  cfblk4/1 -> cfblk18/1
  cfblk18/1 -> cfblk3/1
  cfblk12/1(cfblk2) -> cfblk19/1
  cfblk19/1 -> cfblk5/1

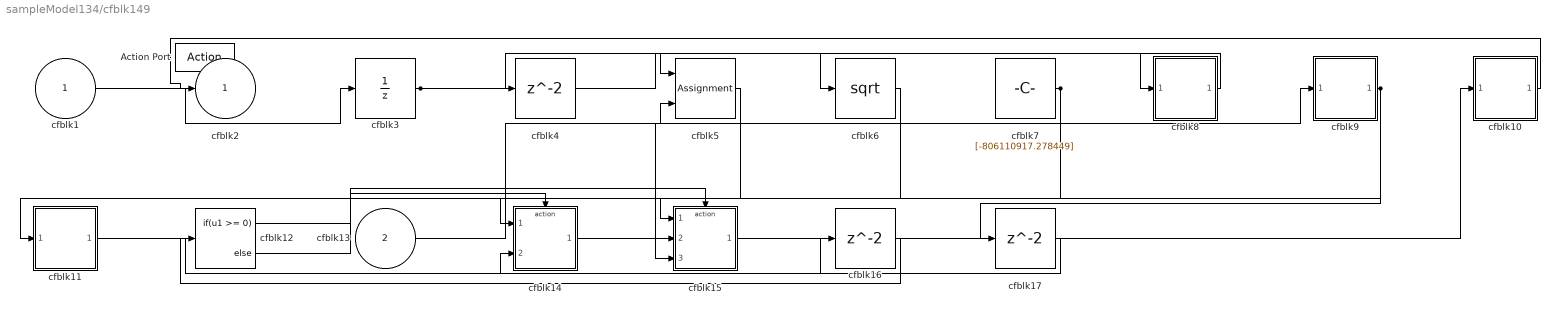
== system sampleModel134/cfblk149 ==
  cfblk1 : Inport
  cfblk13 : Inport  Port=2
  Action Port : ActionPort  ActionType=then
  cfblk10 : Subsystem
  cfblk11 : Subsystem
  cfblk12 : If  IfExpression=u1 >= 0  SampleTime=1
  cfblk14 : Subsystem  TreatAsAtomicUnit=on
  cfblk15 : Subsystem  TreatAsAtomicUnit=on
  cfblk16 : Delay
  cfblk17 : Delay
  cfblk3 : UnitDelay  SampleTime=-1
  cfblk4 : Delay
  cfblk5 : Assignment  DiagnosticForDimensions=Warning  IndexOptions=Index vector (dialog)  Indices=1  OutputSizes=1
  cfblk6 : Sqrt  SaturateOnIntegerOverflow=on
  cfblk7 : Constant  Value=[-806110917.278449]  SampleTime=1
  cfblk8 : Subsystem
  cfblk9 : Subsystem
  cfblk2 : Outport
  wires:
  cfblk9/1(cfblk2) -> cfblk11/1(cfblk1), cfblk17/1
  cfblk3/1 -> cfblk5/1, cfblk4/1
  cfblk8/1(cfblk2) -> cfblk6/1
  cfblk13/1 -> cfblk5/2
  cfblk7/1 -> cfblk15/1(cfblk1), cfblk14/1(cfblk1)
  cfblk1/1 -> cfblk3/1
  cfblk5/1 -> cfblk15/2(cfblk16)
  cfblk4/1 -> cfblk8/1(cfblk1)
  cfblk15/1(cfblk2) -> cfblk10/1(cfblk1)
  cfblk10/1(cfblk2) -> cfblk2/1
  cfblk6/1 -> cfblk15/3(cfblk17)
  cfblk14/1(cfblk2) -> cfblk9/1(cfblk1)
  cfblk12/1 -> cfblk14/Action
  cfblk12/2 -> cfblk15/Action
  cfblk11/1(cfblk2) -> cfblk16/1
  cfblk16/1 -> cfblk12/1
  cfblk17/1 -> cfblk14/2(cfblk12)

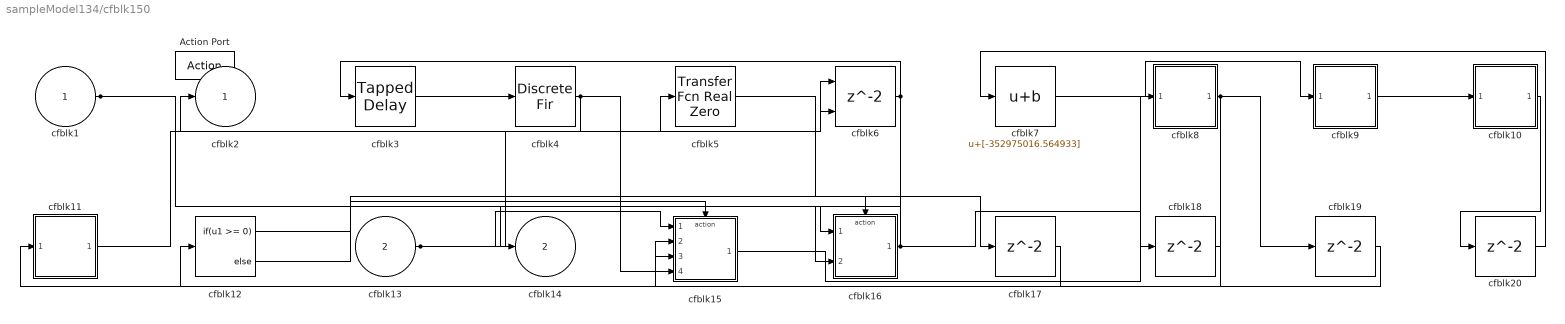
== system sampleModel134/cfblk150 ==
  cfblk1 : Inport
  cfblk13 : Inport  Port=2
  Action Port : ActionPort  ActionType=else
  cfblk10 : Subsystem
  cfblk11 : Subsystem
  cfblk12 : If  IfExpression=u1 >= 0  SampleTime=1
  cfblk15 : Subsystem  TreatAsAtomicUnit=on
  cfblk16 : Subsystem  TreatAsAtomicUnit=on
  cfblk{17..20} (4 alike) : Delay
  cfblk3 : simulink/Discrete/Tapped Delay  vinit=0.0  samptime=-1  NumDelays=1  DelayOrder=Oldest  includeCurrent=off
  cfblk4 : DiscreteFir
  cfblk5 : simulink/Discrete/Transfer Fcn Real Zero  ZeroZ=0.75  ICPrevInput=0.0  DoSatur=off
      settings: SourceProductName=Simulink  SourceProductBaseCode=SL
  cfblk6 : Delay  ShowEnablePort=on
      settings: InputPortMap=u0,e6
  cfblk7 : Bias  Bias=[-352975016.564933]
  cfblk8 : Subsystem
  cfblk9 : Subsystem
  cfblk2 : Outport
  cfblk14 : Outport  Port=2
  wires:
  cfblk6/1 -> cfblk3/1, cfblk16/2(cfblk11)
  cfblk3/1 -> cfblk4/1
  cfblk9/1(cfblk2) -> cfblk10/1(cfblk1)
  cfblk8/1(cfblk2) -> cfblk11/1(cfblk1), cfblk19/1
  cfblk7/1 -> cfblk9/1(cfblk1)
  cfblk11/1(cfblk2) -> cfblk5/1
  cfblk13/1 -> cfblk6/1, cfblk15/1(cfblk1)
  cfblk4/1 -> cfblk2/1, cfblk15/4(cfblk17)
  cfblk16/1(cfblk2) -> cfblk14/1, cfblk18/1
  cfblk15/1(cfblk2) -> cfblk8/1(cfblk1)
  cfblk1/1 -> cfblk6/2, cfblk16/1(cfblk1)
  cfblk12/1 -> cfblk15/Action
  cfblk12/2 -> cfblk16/Action
  cfblk5/1 -> cfblk17/1
  cfblk17/1 -> cfblk12/1
  cfblk18/1 -> cfblk15/2(cfblk15)
  cfblk19/1 -> cfblk15/3(cfblk16)
  cfblk10/1(cfblk2) -> cfblk20/1
  cfblk20/1 -> cfblk7/1

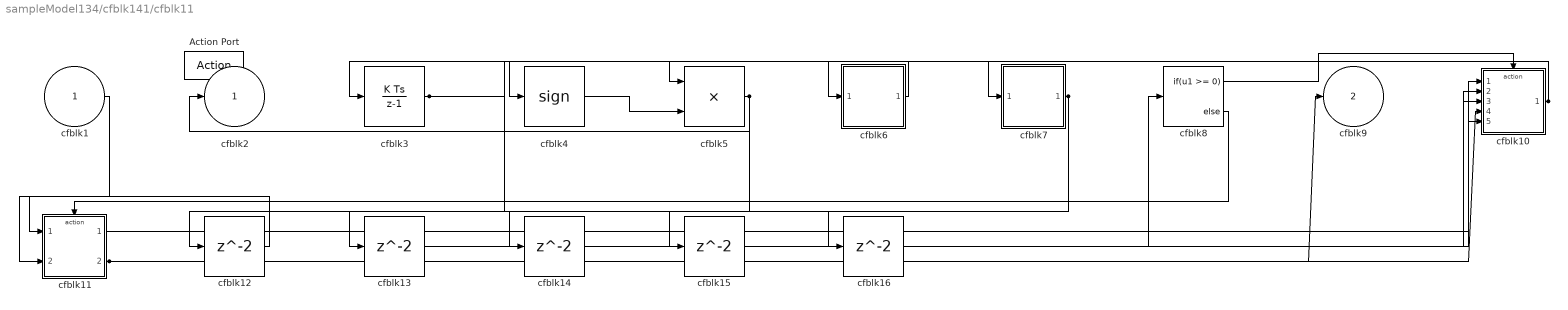
== system sampleModel134/cfblk141/cfblk11 ==
  cfblk1 : Inport
  Action Port : ActionPort  ActionType=then
  cfblk10 : Subsystem  TreatAsAtomicUnit=on
  cfblk11 : Subsystem  TreatAsAtomicUnit=on
  cfblk{12..16} (5 alike) : Delay
  cfblk3 : DiscreteIntegrator  SampleTime=-1  ICPrevOutput=DiscIntNeverNeededParam  ICPrevScaledInput=DiscIntNeverNeededParam
  cfblk4 : Signum
  cfblk5 : Product
  cfblk6 : Subsystem
  cfblk7 : Subsystem
  cfblk8 : If  IfExpression=u1 >= 0  SampleTime=1
  cfblk2 : Outport
  cfblk9 : Outport  Port=2
  wires:
  cfblk5/1 -> cfblk2/1, cfblk14/1, cfblk15/1
  cfblk11/1(cfblk2) -> cfblk10/1(cfblk1)
  cfblk6/1(cfblk2) -> cfblk4/1
  cfblk7/1(cfblk2) -> cfblk12/1, cfblk13/1
  cfblk10/1(cfblk2) -> cfblk7/1(cfblk1), cfblk3/1, cfblk6/1(cfblk1)
  cfblk11/2(cfblk8) -> cfblk9/1, cfblk10/4(cfblk16)
  cfblk1/1 -> cfblk11/2(cfblk7)
  cfblk3/1 -> cfblk5/1, cfblk16/1
  cfblk4/1 -> cfblk5/2
  cfblk8/1 -> cfblk10/Action
  cfblk8/2 -> cfblk11/Action
  cfblk12/1 -> cfblk11/1(cfblk1)
  cfblk13/1 -> cfblk8/1
  cfblk14/1 -> cfblk10/3(cfblk15)
  cfblk15/1 -> cfblk10/5(cfblk17)
  cfblk16/1 -> cfblk10/2(cfblk14)

== system sampleModel134/cfblk141/cfblk12 ==
  cfblk1 : Inport
  cfblk8 : Inport  Port=2
  Action Port : ActionPort  ActionType=else
  cfblk3 : DotProduct  InputSameDT=on  OutDataTypeStr=Inherit: Inherit via internal rule
  cfblk4 : Sum  Inputs=+-
  cfblk5 : Constant  Value=[-9028044.200234]  SampleTime=1
  cfblk6 : Subsystem
  cfblk7 : Subsystem
  cfblk9 : Delay
  cfblk2 : Outport
  wires:
  cfblk6/1(cfblk2) -> cfblk7/1(cfblk1)
  cfblk1/1 -> cfblk4/1
  cfblk4/1 -> cfblk3/1
  cfblk5/1 -> cfblk3/2
  cfblk3/1 -> cfblk2/1
  cfblk8/1 -> cfblk4/2
  cfblk7/1(cfblk2) -> cfblk9/1
  cfblk9/1 -> cfblk6/1(cfblk1)

== system sampleModel134/cfblk141/cfblk5 ==
  cfblk1 : Inport
  cfblk2 : Outport
  wires:
  cfblk1/1 -> cfblk2/1

== system sampleModel134/cfblk141/cfblk6 ==
  cfblk1 : Inport
  cfblk2 : Outport
  wires:
  cfblk1/1 -> cfblk2/1

== system sampleModel134/cfblk141/cfblk7 ==
  cfblk1 : Inport
  cfblk2 : Outport
  wires:
  cfblk1/1 -> cfblk2/1

== system sampleModel134/cfblk141/cfblk8 ==
  cfblk1 : Inport
  cfblk2 : Outport
  wires:
  cfblk1/1 -> cfblk2/1

== system sampleModel134/cfblk142/cfblk11 ==
  cfblk1 : Inport
  cfblk2 : Outport
  wires:
  cfblk1/1 -> cfblk2/1

== system sampleModel134/cfblk144/cfblk11 ==
  cfblk1 : Inport
  cfblk2 : Outport
  wires:
  cfblk1/1 -> cfblk2/1

== system sampleModel134/cfblk144/cfblk12 ==
  cfblk1 : Inport
  cfblk2 : Outport
  wires:
  cfblk1/1 -> cfblk2/1

== system sampleModel134/cfblk144/cfblk13 ==
  cfblk1 : Inport
  cfblk2 : Outport
  wires:
  cfblk1/1 -> cfblk2/1

== system sampleModel134/cfblk145/cfblk4 ==
  cfblk1 : Inport
  cfblk2 : Outport
  wires:
  cfblk1/1 -> cfblk2/1

== system sampleModel134/cfblk145/cfblk5 ==
  cfblk1 : Inport
  cfblk2 : Outport
  wires:
  cfblk1/1 -> cfblk2/1

== system sampleModel134/cfblk145/cfblk6 ==
  cfblk1 : Inport
  cfblk2 : Outport
  wires:
  cfblk1/1 -> cfblk2/1

== system sampleModel134/cfblk145/cfblk7 ==
  cfblk1 : Inport
  cfblk2 : Outport
  wires:
  cfblk1/1 -> cfblk2/1

== system sampleModel134/cfblk146/cfblk10 ==
  cfblk1 : Inport
  cfblk2 : Outport
  wires:
  cfblk1/1 -> cfblk2/1

== system sampleModel134/cfblk146/cfblk11 ==
  cfblk1 : Inport
  cfblk2 : Outport
  wires:
  cfblk1/1 -> cfblk2/1

== system sampleModel134/cfblk146/cfblk12 ==
  cfblk1 : Inport
  cfblk2 : Outport
  wires:
  cfblk1/1 -> cfblk2/1

== system sampleModel134/cfblk146/cfblk13 ==
  cfblk1 : Inport
  cfblk2 : Outport
  wires:
  cfblk1/1 -> cfblk2/1

== system sampleModel134/cfblk147/cfblk4 ==
  cfblk1 : Inport
  cfblk2 : Outport
  wires:
  cfblk1/1 -> cfblk2/1

== system sampleModel134/cfblk148/cfblk10 ==
  cfblk1 : Inport
  cfblk2 : Outport
  wires:
  cfblk1/1 -> cfblk2/1

== system sampleModel134/cfblk148/cfblk11 ==
  cfblk1 : Inport
  cfblk2 : Outport
  wires:
  cfblk1/1 -> cfblk2/1

== system sampleModel134/cfblk148/cfblk12 ==
  cfblk1 : Inport
  cfblk2 : Outport
  wires:
  cfblk1/1 -> cfblk2/1

== system sampleModel134/cfblk148/cfblk13 ==
  cfblk1 : Inport
  cfblk2 : Outport
  wires:
  cfblk1/1 -> cfblk2/1

== system sampleModel134/cfblk148/cfblk14 ==
  cfblk1 : Inport
  cfblk2 : Outport
  wires:
  cfblk1/1 -> cfblk2/1

== system sampleModel134/cfblk148/cfblk7 ==
  cfblk1 : Inport
  cfblk2 : Outport
  wires:
  cfblk1/1 -> cfblk2/1

== system sampleModel134/cfblk148/cfblk8 ==
  cfblk1 : Inport
  cfblk2 : Outport
  wires:
  cfblk1/1 -> cfblk2/1

== system sampleModel134/cfblk148/cfblk9 ==
  cfblk1 : Inport
  cfblk2 : Outport
  wires:
  cfblk1/1 -> cfblk2/1

== system sampleModel134/cfblk149/cfblk10 ==
  cfblk1 : Inport
  cfblk2 : Outport
  wires:
  cfblk1/1 -> cfblk2/1

== system sampleModel134/cfblk149/cfblk11 ==
  cfblk1 : Inport
  cfblk2 : Outport
  wires:
  cfblk1/1 -> cfblk2/1

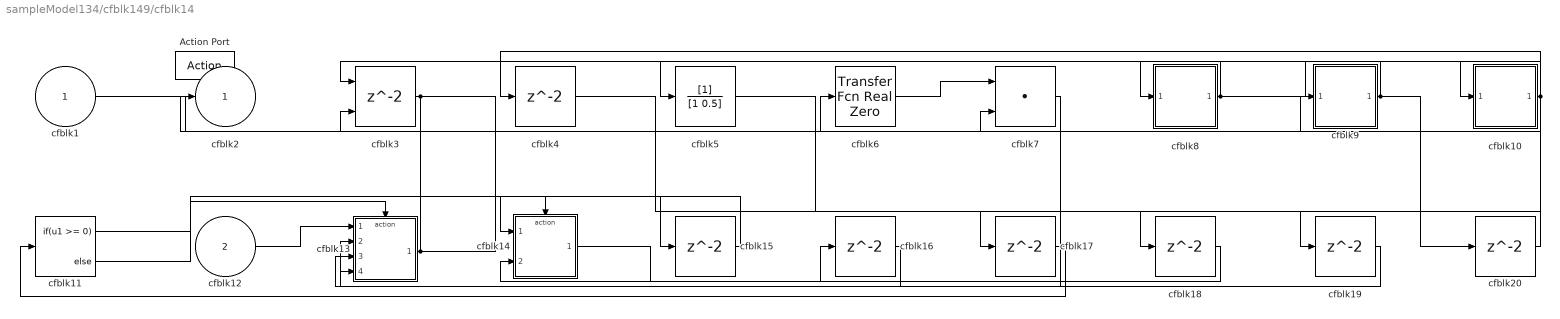
== system sampleModel134/cfblk149/cfblk14 ==
  cfblk1 : Inport
  cfblk12 : Inport  Port=2
  Action Port : ActionPort  ActionType=then
  cfblk10 : Subsystem
  cfblk11 : If  IfExpression=u1 >= 0  SampleTime=1
  cfblk13 : Subsystem  TreatAsAtomicUnit=on
  cfblk14 : Subsystem  TreatAsAtomicUnit=on
  cfblk{4,15..20} (7 alike) : Delay
  cfblk3 : Delay  ShowEnablePort=on
      settings: InputPortMap=u0,e6
  cfblk5 : DiscreteFilter
  cfblk6 : simulink/Discrete/Transfer Fcn Real Zero  ZeroZ=0.75  ICPrevInput=0.0  DoSatur=off
      settings: SourceProductName=Simulink  SourceProductBaseCode=SL
  cfblk7 : DotProduct  InputSameDT=on  OutDataTypeStr=Inherit: Inherit via internal rule
  cfblk8 : Subsystem
  cfblk9 : Subsystem
  cfblk2 : Outport
  wires:
  cfblk12/1 -> cfblk13/1(cfblk1)
  cfblk9/1(cfblk2) -> cfblk8/1(cfblk1), cfblk20/1
  cfblk10/1(cfblk2) -> cfblk4/1, cfblk5/1, cfblk18/1
  cfblk7/1 -> cfblk13/2(cfblk11)
  cfblk1/1 -> cfblk6/1
  cfblk8/1(cfblk2) -> cfblk3/1, cfblk10/1(cfblk1)
  cfblk6/1 -> cfblk7/1
  cfblk13/1(cfblk2) -> cfblk3/2, cfblk9/1(cfblk1)
  cfblk3/1 -> cfblk2/1, cfblk15/1
  cfblk11/1 -> cfblk13/Action
  cfblk11/2 -> cfblk14/Action
  cfblk15/1 -> cfblk14/1(cfblk1)
  cfblk14/1(cfblk2) -> cfblk16/1
  cfblk16/1 -> cfblk13/3(cfblk12)
  cfblk4/1 -> cfblk17/1
  cfblk17/1 -> cfblk11/1
  cfblk18/1 -> cfblk14/2(cfblk17)
  cfblk5/1 -> cfblk19/1
  cfblk19/1 -> cfblk13/4(cfblk13)
  cfblk20/1 -> cfblk7/2

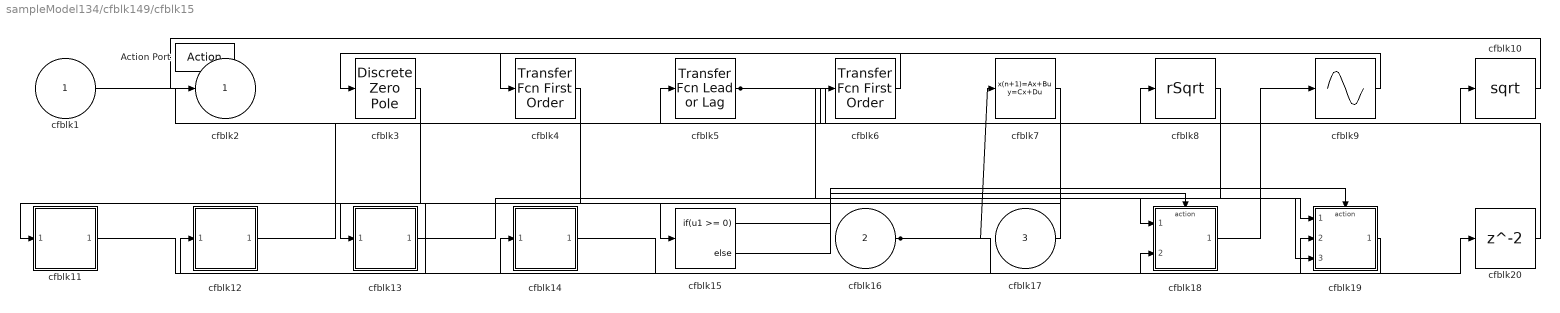
== system sampleModel134/cfblk149/cfblk15 ==
  cfblk1 : Inport
  cfblk16 : Inport  Port=2
  cfblk17 : Inport  Port=3
  Action Port : ActionPort  ActionType=else
  cfblk10 : Sqrt  SaturateOnIntegerOverflow=on
  cfblk11 : Subsystem
  cfblk12 : Subsystem
  cfblk13 : Subsystem
  cfblk14 : Subsystem
  cfblk15 : If  IfExpression=u1 >= 0  SampleTime=1
  cfblk18 : Subsystem  TreatAsAtomicUnit=on
  cfblk19 : Subsystem  TreatAsAtomicUnit=on
  cfblk20 : Delay
  cfblk3 : DiscreteZeroPole  Poles=[0 0.5]  Gain=1  SampleTime=-1
  cfblk4 : simulink/Discrete/Transfer Fcn First Order  PoleZ=0.95  ICPrevOutput=0.0  DoSatur=off
      settings: SourceProductName=Simulink
  cfblk5 : simulink/Discrete/Transfer Fcn Lead or Lag  PoleZ=0.95  ZeroZ=0.75  ICPrevOutput=0.0  ICPrevInput=0.0  DoSatur=off
      settings: SourceProductName=Simulink  SourceProductBaseCode=SL
  cfblk6 : simulink/Discrete/Transfer Fcn First Order  PoleZ=0.95  ICPrevOutput=0.0  DoSatur=off
      settings: SourceProductName=Simulink
  cfblk7 : DiscreteStateSpace  SampleTime=-1
  cfblk8 : Sqrt  Operator=rSqrt  AlgorithmType=Newton-Raphson  SaturateOnIntegerOverflow=on
  cfblk9 : Sin  TimeSource=Use external signal  SampleTime=0
  cfblk2 : Outport
  wires:
  cfblk6/1 -> cfblk3/1
  cfblk5/1 -> cfblk8/1, cfblk19/3(cfblk9)
  cfblk3/1 -> cfblk11/1(cfblk1)
  cfblk4/1 -> cfblk12/1(cfblk1)
  cfblk7/1 -> cfblk13/1(cfblk1)
  cfblk18/1(cfblk2) -> cfblk9/1
  cfblk10/1 -> cfblk2/1
  cfblk12/1(cfblk2) -> cfblk10/1
  cfblk19/1(cfblk2) -> cfblk14/1(cfblk1)
  cfblk8/1 -> cfblk18/1(cfblk1)
  cfblk17/1 -> cfblk15/1
  cfblk9/1 -> cfblk4/1
  cfblk13/1(cfblk2) -> cfblk19/1(cfblk1)
  cfblk11/1(cfblk2) -> cfblk18/2(cfblk11)
  cfblk1/1 -> cfblk6/1
  cfblk16/1 -> cfblk7/1, cfblk19/2(cfblk8)
  cfblk15/1 -> cfblk18/Action
  cfblk15/2 -> cfblk19/Action
  cfblk14/1(cfblk2) -> cfblk20/1
  cfblk20/1 -> cfblk5/1

== system sampleModel134/cfblk149/cfblk8 ==
  cfblk1 : Inport
  cfblk2 : Outport
  wires:
  cfblk1/1 -> cfblk2/1

== system sampleModel134/cfblk149/cfblk9 ==
  cfblk1 : Inport
  cfblk2 : Outport
  wires:
  cfblk1/1 -> cfblk2/1

== system sampleModel134/cfblk150/cfblk10 ==
  cfblk1 : Inport
  cfblk2 : Outport
  wires:
  cfblk1/1 -> cfblk2/1

== system sampleModel134/cfblk150/cfblk11 ==
  cfblk1 : Inport
  cfblk2 : Outport
  wires:
  cfblk1/1 -> cfblk2/1

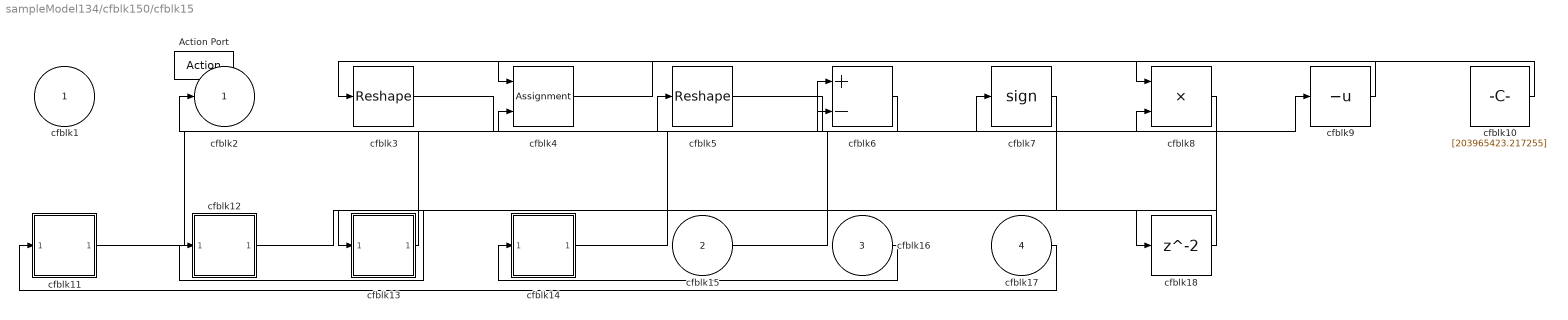
== system sampleModel134/cfblk150/cfblk15 ==
  cfblk1 : Inport
  cfblk15 : Inport  Port=2
  cfblk16 : Inport  Port=3
  cfblk17 : Inport  Port=4
  Action Port : ActionPort  ActionType=then
  cfblk10 : Constant  Value=[203965423.217255]  SampleTime=1
  cfblk11 : Subsystem
  cfblk12 : Subsystem
  cfblk13 : Subsystem
  cfblk14 : Subsystem
  cfblk18 : Delay
  cfblk3 : Reshape
  cfblk4 : Assignment  DiagnosticForDimensions=Warning  IndexOptions=Index vector (dialog)  Indices=1  OutputSizes=1
  cfblk5 : Reshape
  cfblk6 : Sum  Inputs=+-
  cfblk7 : Signum
  cfblk8 : Product  Inputs=**
  cfblk9 : UnaryMinus
  cfblk2 : Outport
  wires:
  cfblk10/1 -> cfblk3/1
  cfblk11/1(cfblk2) -> cfblk6/1
  cfblk9/1 -> cfblk4/1
  cfblk13/1(cfblk2) -> cfblk2/1
  cfblk7/1 -> cfblk12/1(cfblk1)
  cfblk5/1 -> cfblk7/1
  cfblk4/1 -> cfblk8/1
  cfblk6/1 -> cfblk4/2
  cfblk16/1 -> cfblk14/1(cfblk1)
  cfblk8/1 -> cfblk13/1(cfblk1)
  cfblk14/1(cfblk2) -> cfblk8/2
  cfblk3/1 -> cfblk6/2
  cfblk15/1 -> cfblk9/1
  cfblk17/1 -> cfblk11/1(cfblk1)
  cfblk12/1(cfblk2) -> cfblk18/1
  cfblk18/1 -> cfblk5/1

== system sampleModel134/cfblk150/cfblk16 ==
  cfblk1 : Inport
  cfblk11 : Inport  Port=2
  Action Port : ActionPort  ActionType=else
  cfblk10 : Subsystem
  cfblk12 : Delay
  cfblk13 : Delay
  cfblk14 : Delay
  cfblk3 : simulink/Discrete/Tapped Delay  vinit=0.0  samptime=-1  NumDelays=1  DelayOrder=Oldest  includeCurrent=off
  cfblk4 : simulink/Discrete/Transfer Fcn Real Zero  ZeroZ=0.75  ICPrevInput=0.0  DoSatur=off
      settings: SourceProductName=Simulink  SourceProductBaseCode=SL
  cfblk5 : simulink/Discrete/Transfer Fcn Real Zero  ZeroZ=0.75  ICPrevInput=0.0  DoSatur=off
      settings: SourceProductName=Simulink  SourceProductBaseCode=SL
  cfblk6 : Product  Inputs=**
  cfblk7 : Subsystem
  cfblk8 : Subsystem
  cfblk9 : Subsystem
  cfblk2 : Outport
  wires:
  cfblk6/1 -> cfblk9/1(cfblk1)
  cfblk4/1 -> cfblk10/1(cfblk1)
  cfblk11/1 -> cfblk8/1(cfblk1)
  cfblk8/1(cfblk2) -> cfblk5/1
  cfblk1/1 -> cfblk6/2
  cfblk3/1 -> cfblk7/1(cfblk1)
  cfblk5/1 -> cfblk2/1
  cfblk9/1(cfblk2) -> cfblk12/1
  cfblk12/1 -> cfblk6/1
  cfblk7/1(cfblk2) -> cfblk13/1
  cfblk13/1 -> cfblk3/1
  cfblk10/1(cfblk2) -> cfblk14/1
  cfblk14/1 -> cfblk4/1

== system sampleModel134/cfblk150/cfblk8 ==
  cfblk1 : Inport
  cfblk2 : Outport
  wires:
  cfblk1/1 -> cfblk2/1

== system sampleModel134/cfblk150/cfblk9 ==
  cfblk1 : Inport
  cfblk2 : Outport
  wires:
  cfblk1/1 -> cfblk2/1

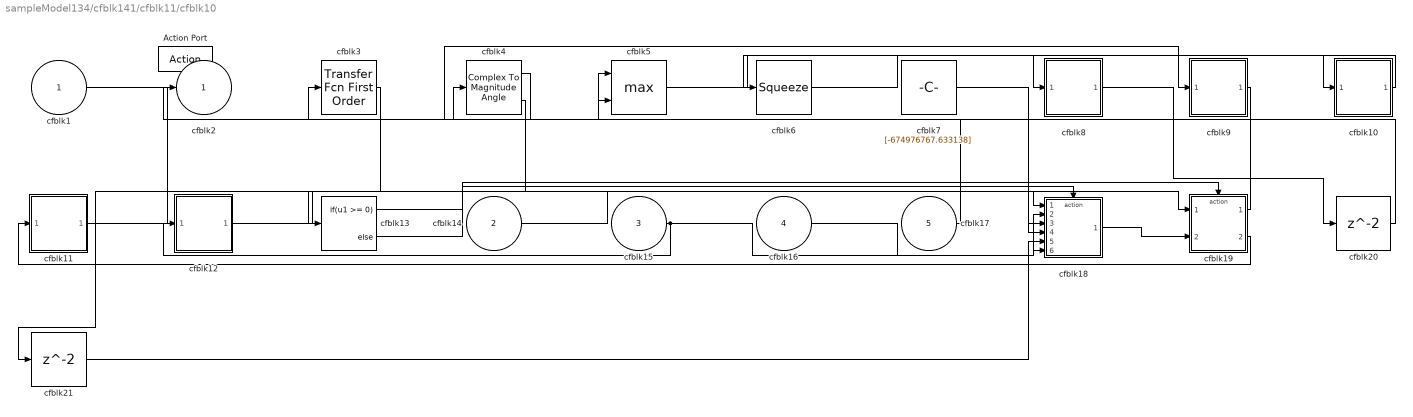
== system sampleModel134/cfblk141/cfblk11/cfblk10 ==
  cfblk1 : Inport
  cfblk14 : Inport  Port=2
  cfblk15 : Inport  Port=3
  cfblk16 : Inport  Port=4
  cfblk17 : Inport  Port=5
  Action Port : ActionPort  ActionType=then
  cfblk10 : Subsystem
  cfblk11 : Subsystem
  cfblk12 : Subsystem
  cfblk13 : If  IfExpression=u1 >= 0  SampleTime=1
  cfblk18 : Subsystem  TreatAsAtomicUnit=on
  cfblk19 : Subsystem  TreatAsAtomicUnit=on
  cfblk20 : Delay
  cfblk21 : Delay
  cfblk3 : simulink/Discrete/Transfer Fcn First Order  PoleZ=0.95  ICPrevOutput=0.0  DoSatur=off
      settings: SourceProductName=Simulink
  cfblk4 : ComplexToMagnitudeAngle
  cfblk5 : MinMax  Function=max  Inputs=2
  cfblk6 : Squeeze
  cfblk7 : Constant  Value=[-674976767.633138]  SampleTime=1
  cfblk8 : Subsystem
  cfblk9 : Subsystem
  cfblk2 : Outport
  wires:
  cfblk6/1 -> cfblk8/1(cfblk1)
  cfblk9/1(cfblk2) -> cfblk4/1
  cfblk12/1(cfblk2) -> cfblk18/1(cfblk1)
  cfblk11/1(cfblk2) -> cfblk9/1(cfblk1)
  cfblk5/1 -> cfblk10/1(cfblk1)
  cfblk15/1 -> cfblk12/1(cfblk1), cfblk18/6(cfblk14)
  cfblk16/1 -> cfblk18/2(cfblk10)
  cfblk10/1(cfblk2) -> cfblk6/1
  cfblk14/1 -> cfblk18/3(cfblk11)
  cfblk3/1 -> cfblk13/1
  cfblk1/1 -> cfblk18/4(cfblk12)
  cfblk7/1 -> cfblk19/1(cfblk1)
  cfblk19/1(cfblk2) -> cfblk5/1
  cfblk4/1 -> cfblk2/1
  cfblk18/1(cfblk2) -> cfblk19/2(cfblk13)
  cfblk17/1 -> cfblk3/1
  cfblk19/2(cfblk14) -> cfblk11/1(cfblk1)
  cfblk13/1 -> cfblk18/Action
  cfblk13/2 -> cfblk19/Action
  cfblk8/1(cfblk2) -> cfblk20/1
  cfblk20/1 -> cfblk5/2
  cfblk4/2 -> cfblk21/1
  cfblk21/1 -> cfblk18/5(cfblk13)

== system sampleModel134/cfblk141/cfblk11/cfblk11 ==
  cfblk1 : Inport
  cfblk7 : Inport  Port=2
  Action Port : ActionPort  ActionType=else
  cfblk10 : Subsystem  TreatAsAtomicUnit=on
  cfblk11 : Delay
  cfblk12 : Delay
  cfblk3 : Assignment  DiagnosticForDimensions=Warning  IndexOptions=Index vector (dialog)  Indices=1  OutputSizes=1
  cfblk4 : Subsystem
  cfblk5 : Subsystem
  cfblk6 : If  IfExpression=u1 >= 0  SampleTime=1
  cfblk9 : Subsystem  TreatAsAtomicUnit=on
  cfblk2 : Outport
  cfblk8 : Outport  Port=2
  wires:
  cfblk9/1(cfblk2) -> cfblk4/1(cfblk1)
  cfblk10/1(cfblk2) -> cfblk5/1(cfblk1)
  cfblk7/1 -> cfblk6/1
  cfblk3/1 -> cfblk9/2(cfblk8)
  cfblk9/2(cfblk10) -> cfblk8/1
  cfblk10/2(cfblk8) -> cfblk9/3(cfblk9)
  cfblk1/1 -> cfblk3/2, cfblk10/1(cfblk1), cfblk10/2(cfblk7)
  cfblk10/3(cfblk9) -> cfblk2/1
  cfblk6/1 -> cfblk9/Action
  cfblk6/2 -> cfblk10/Action
  cfblk4/1(cfblk2) -> cfblk11/1
  cfblk11/1 -> cfblk3/1
  cfblk5/1(cfblk2) -> cfblk12/1
  cfblk12/1 -> cfblk9/1(cfblk1)

== system sampleModel134/cfblk141/cfblk11/cfblk6 ==
  cfblk1 : Inport
  cfblk2 : Outport
  wires:
  cfblk1/1 -> cfblk2/1

== system sampleModel134/cfblk141/cfblk11/cfblk7 ==
  cfblk1 : Inport
  cfblk2 : Outport
  wires:
  cfblk1/1 -> cfblk2/1

== system sampleModel134/cfblk141/cfblk12/cfblk6 ==
  cfblk1 : Inport
  cfblk2 : Outport
  wires:
  cfblk1/1 -> cfblk2/1

== system sampleModel134/cfblk141/cfblk12/cfblk7 ==
  cfblk1 : Inport
  cfblk2 : Outport
  wires:
  cfblk1/1 -> cfblk2/1

== system sampleModel134/cfblk149/cfblk14/cfblk10 ==
  cfblk1 : Inport
  cfblk2 : Outport
  wires:
  cfblk1/1 -> cfblk2/1

== system sampleModel134/cfblk149/cfblk14/cfblk13 ==
  cfblk1 : Inport
  cfblk11 : Inport  Port=2
  cfblk12 : Inport  Port=3
  cfblk13 : Inport  Port=4
  Action Port : ActionPort  ActionType=then
  cfblk10 : Subsystem
  cfblk3 : simulink/Discrete/Transfer Fcn Lead or Lag  PoleZ=0.95  ZeroZ=0.75  ICPrevOutput=0.0  ICPrevInput=0.0  DoSatur=off
      settings: SourceProductName=Simulink  SourceProductBaseCode=SL
  cfblk4 : simulink/Discrete/Transfer Fcn Lead or Lag  PoleZ=0.95  ZeroZ=0.75  ICPrevOutput=0.0  ICPrevInput=0.0  DoSatur=off
      settings: SourceProductName=Simulink  SourceProductBaseCode=SL
  cfblk5 : Gain  Gain=[-226698156.817862]
  cfblk6 : Polyval  Coefs=[ +2.081618890e-019, -1.441693666e-014, +4.719686976e-010, -8.536869453e-006, +1.621573104e-001, -8.087801117e+001 ]
  cfblk7 : Constant  Value=[698115365.988320]  SampleTime=1
  cfblk8 : Subsystem
  cfblk9 : Subsystem
  cfblk2 : Outport
  wires:
  cfblk13/1 -> cfblk9/1(cfblk1)
  cfblk8/1(cfblk2) -> cfblk4/1
  cfblk12/1 -> cfblk6/1
  cfblk6/1 -> cfblk3/1
  cfblk9/1(cfblk2) -> cfblk10/1(cfblk1)
  cfblk3/1 -> cfblk5/1
  cfblk11/1 -> cfblk8/1(cfblk1)
  cfblk1/1 -> cfblk2/1

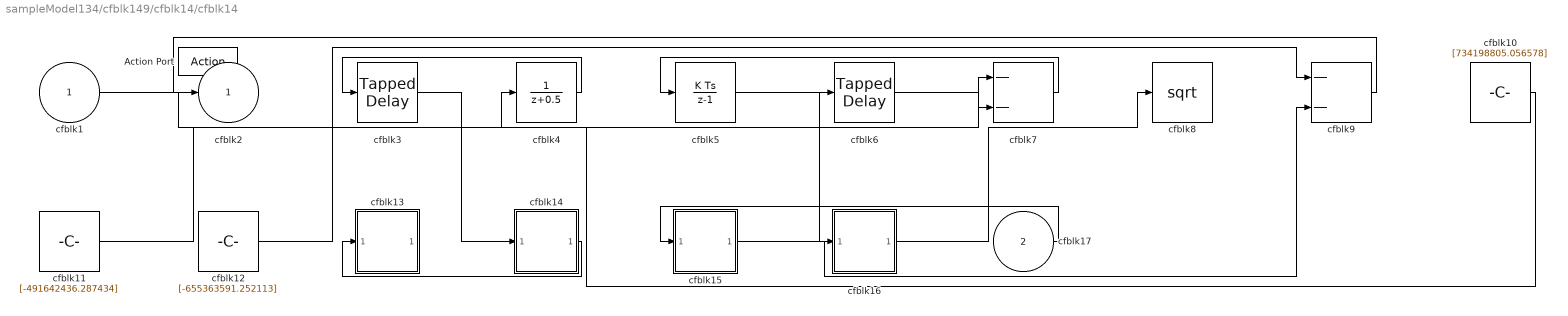
== system sampleModel134/cfblk149/cfblk14/cfblk14 ==
  cfblk1 : Inport
  cfblk17 : Inport  Port=2
  Action Port : ActionPort  ActionType=else
  cfblk10 : Constant  Value=[734198805.056578]  SampleTime=1
  cfblk11 : Constant  Value=[-491642436.287434]  SampleTime=1
  cfblk12 : Constant  Value=[-655363591.252113]  SampleTime=1
  cfblk13 : Subsystem
  cfblk14 : Subsystem
  cfblk15 : Subsystem
  cfblk16 : Subsystem
  cfblk3 : simulink/Discrete/Tapped Delay  vinit=0.0  samptime=-1  NumDelays=1  DelayOrder=Oldest  includeCurrent=off
  cfblk4 : DiscreteTransferFcn
  cfblk5 : DiscreteIntegrator  SampleTime=-1  ICPrevOutput=DiscIntNeverNeededParam  ICPrevScaledInput=DiscIntNeverNeededParam
  cfblk6 : simulink/Discrete/Tapped Delay  vinit=0.0  samptime=-1  NumDelays=1  DelayOrder=Oldest  includeCurrent=off
  cfblk7 : Sum  Inputs=--
  cfblk8 : Sqrt  SaturateOnIntegerOverflow=on
  cfblk9 : Sum  Inputs=--
  cfblk2 : Outport
  wires:
  cfblk3/1 -> cfblk14/1(cfblk1)
  cfblk4/1 -> cfblk3/1
  cfblk12/1 -> cfblk9/1
  cfblk17/1 -> cfblk15/1(cfblk1)
  cfblk15/1(cfblk2) -> cfblk9/2
  cfblk16/1(cfblk2) -> cfblk8/1
  cfblk5/1 -> cfblk16/1(cfblk1)
  cfblk7/1 -> cfblk5/1
  cfblk9/1 -> cfblk2/1
  cfblk10/1 -> cfblk4/1
  cfblk14/1(cfblk2) -> cfblk13/1(cfblk1)
  cfblk1/1 -> cfblk7/1
  cfblk11/1 -> cfblk6/1
  cfblk6/1 -> cfblk7/2

== system sampleModel134/cfblk149/cfblk14/cfblk8 ==
  cfblk1 : Inport
  cfblk2 : Outport
  wires:
  cfblk1/1 -> cfblk2/1

== system sampleModel134/cfblk149/cfblk14/cfblk9 ==
  cfblk1 : Inport
  cfblk2 : Outport
  wires:
  cfblk1/1 -> cfblk2/1

== system sampleModel134/cfblk149/cfblk15/cfblk11 ==
  cfblk1 : Inport
  cfblk2 : Outport
  wires:
  cfblk1/1 -> cfblk2/1
